simulink model "Stepper2"  (Simulink 7.6)
settings: Solver=ode45  StartTime=0.0  StopTime=1  RelTol=1e-3
libraries: simulink x13
settings Model: Creator=MTRStudent  LastModifiedBy=Mr_lex
settings DebuggingCC: StrictBusMsg=Warning

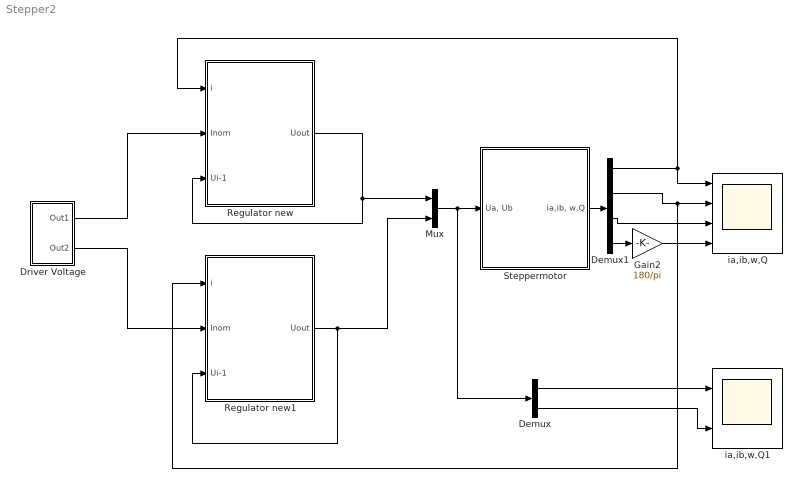
== system Stepper2 ==
  Demux : Demux  Outputs=2
  Demux1 : Demux
  Driver Voltage : Subsystem
  Gain2 : Gain  Gain=180/pi
  Mux : Mux  Inputs=2
  Regulator new : Subsystem
  Regulator new1 : Subsystem
  Steppermotor : Subsystem
  ia,ib,w,Q : Scope  NumInputPorts=4
      settings: TimeRange=0.004  YMin=-0.125~5.875~22~0.7  YMax=0.125~6.125~28.5~2.5  SaveName=ScopeData2
  ia,ib,w,Q1 : Scope  NumInputPorts=2
      settings: YMin=5.45~-2.75  YMax=6.4~1.25
  wires:
  Demux1/1 -> ia,ib,w,Q/1, Regulator new/1(i)
  Demux1/2 -> ia,ib,w,Q/2, Regulator new1/1(i)
  Demux1/3 -> ia,ib,w,Q/3
  Demux1/4 -> Gain2/1
  Steppermotor/1("ia,ib, w,Q") -> Demux1/1
  Mux/1 -> Steppermotor/1("Ua, Ub"), Demux/1
  Demux/1 -> ia,ib,w,Q1/1
  Demux/2 -> ia,ib,w,Q1/2
  Regulator new1/1(Uout) -> Mux/2, Regulator new1/3(Ui-1)
  Regulator new/1(Uout) -> Mux/1, Regulator new/3(Ui-1)
  Gain2/1 -> ia,ib,w,Q/4
  Driver Voltage/1(Out1) -> Regulator new/2(Inom)
  Driver Voltage/2(Out2) -> Regulator new1/2(Inom)

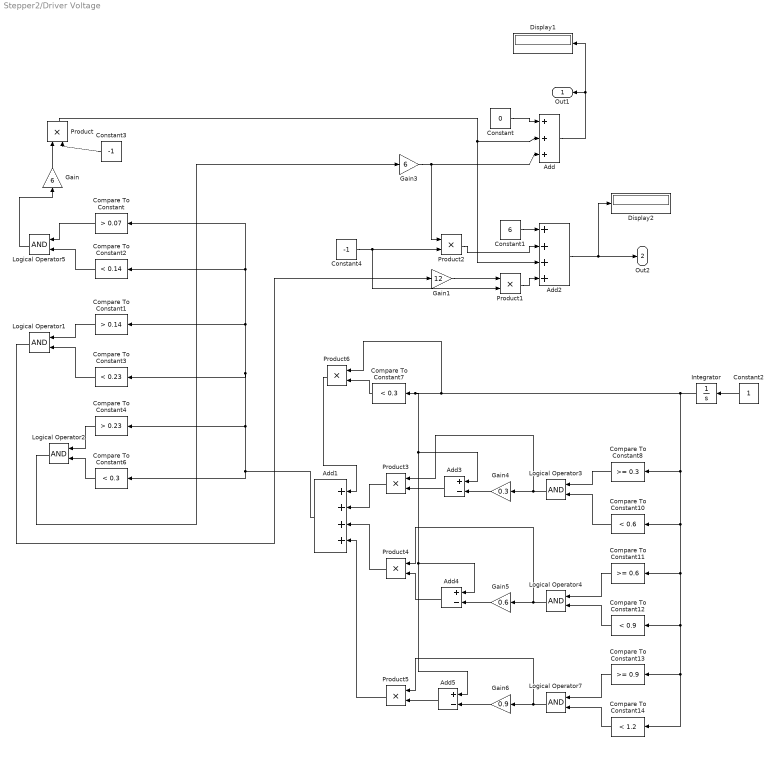
== system Stepper2/Driver Voltage ==
  Add : Sum  Inputs=+++
  Add1 : Sum  Inputs=++++
  Add2 : Sum  Inputs=++++
  Add3 : Sum  Inputs=+-
  Add4 : Sum  Inputs=+-
  Add5 : Sum  Inputs=+-
  Compare To Constant : simulink/Logic and Bit Operations/Compare To Constant  SystemSampleTime=-1  relop=>  const=0.07  LogicOutDataTypeMode=uint8  ZeroCross=off
  Compare To Constant1 : simulink/Logic and Bit Operations/Compare To Constant  SystemSampleTime=-1  relop=>  const=0.14  LogicOutDataTypeMode=uint8  ZeroCross=off
  Compare To Constant10 : simulink/Logic and Bit Operations/Compare To Constant  SystemSampleTime=-1  relop=<  const=0.6  LogicOutDataTypeMode=uint8  ZeroCross=off
  Compare To Constant11 : simulink/Logic and Bit Operations/Compare To Constant  SystemSampleTime=-1  relop=>=  const=0.6  LogicOutDataTypeMode=uint8  ZeroCross=off
  Compare To Constant12 : simulink/Logic and Bit Operations/Compare To Constant  SystemSampleTime=-1  relop=<  const=0.9  LogicOutDataTypeMode=uint8  ZeroCross=off
  Compare To Constant13 : simulink/Logic and Bit Operations/Compare To Constant  SystemSampleTime=-1  relop=>=  const=0.9  LogicOutDataTypeMode=uint8  ZeroCross=off
  Compare To Constant14 : simulink/Logic and Bit Operations/Compare To Constant  SystemSampleTime=-1  relop=<  const=1.2  LogicOutDataTypeMode=uint8  ZeroCross=off
  Compare To Constant2 : simulink/Logic and Bit Operations/Compare To Constant  SystemSampleTime=-1  relop=<  const=0.14  LogicOutDataTypeMode=uint8  ZeroCross=off
  Compare To Constant3 : simulink/Logic and Bit Operations/Compare To Constant  SystemSampleTime=-1  relop=<  const=0.23  LogicOutDataTypeMode=uint8  ZeroCross=off
  Compare To Constant4 : simulink/Logic and Bit Operations/Compare To Constant  SystemSampleTime=-1  relop=>  const=0.23  LogicOutDataTypeMode=uint8  ZeroCross=off
  Compare To Constant6 : simulink/Logic and Bit Operations/Compare To Constant  SystemSampleTime=-1  relop=<  const=0.3  LogicOutDataTypeMode=uint8  ZeroCross=off
  Compare To Constant7 : simulink/Logic and Bit Operations/Compare To Constant  SystemSampleTime=-1  relop=<  const=0.3  LogicOutDataTypeMode=uint8  ZeroCross=off
  Compare To Constant8 : simulink/Logic and Bit Operations/Compare To Constant  SystemSampleTime=-1  relop=>=  const=0.3  LogicOutDataTypeMode=uint8  ZeroCross=off
  Constant : Constant  Value=0
  Constant1 : Constant  Value=6
  Constant2 : Constant
  Constant3 : Constant  Value=-1
  Constant4 : Constant  Value=-1
  Display1 : Display
  Display2 : Display
  Gain : Gain  Gain=6
  Gain1 : Gain  Gain=12
  Gain3 : Gain  Gain=6
  Gain4 : Gain  Gain=0.3
  Gain5 : Gain  Gain=0.6
  Gain6 : Gain  Gain=0.9
  Integrator : Integrator
  Logical Operator{1..5,7} (6 alike) : Logic  AllPortsSameDT=off  OutDataTypeStr=boolean
  Product{,1..6} (7 alike) : Product  RndMeth=Zero
  Out1 : Outport
  Out2 : Outport  Port=2
  wires:
  Add/1 -> Out1/1, Display1/1
  Constant/1 -> Add/1
  Constant1/1 -> Add2/1
  Gain/1 -> Product/1
  Constant3/1 -> Product/2
  Compare To Constant/1 -> Logical Operator5/1
  Compare To Constant2/1 -> Logical Operator5/2
  Logical Operator5/1 -> Gain/1
  Gain1/1 -> Product1/1
  Product1/1 -> Add2/4
  Compare To Constant1/1 -> Logical Operator1/1
  Compare To Constant3/1 -> Logical Operator1/2
  Gain3/1 -> Add/3, Product2/1
  Product2/1 -> Add2/2
  Add2/1 -> Out2/1, Display2/1
  Product/1 -> Add/2, Add2/3
  Constant4/1 -> Product2/2, Product1/2
  Logical Operator1/1 -> Gain1/1
  Compare To Constant4/1 -> Logical Operator2/1
  Compare To Constant6/1 -> Logical Operator2/2
  Logical Operator2/1 -> Gain3/1
  Constant2/1 -> Integrator/1
  Integrator/1 -> Compare To Constant8/1, Compare To Constant10/1, Compare To Constant11/1, Compare To Constant12/1, Compare To Constant13/1, Compare To Constant14/1, Add4/1, Add5/1, Add3/1, Compare To Constant7/1, Product6/1
  Compare To Constant8/1 -> Logical Operator3/1
  Compare To Constant10/1 -> Logical Operator3/2
  Compare To Constant11/1 -> Logical Operator4/1
  Compare To Constant12/1 -> Logical Operator4/2
  Compare To Constant13/1 -> Logical Operator7/1
  Compare To Constant14/1 -> Logical Operator7/2
  Logical Operator3/1 -> Gain4/1, Product3/1
  Logical Operator4/1 -> Gain5/1, Product4/1
  Logical Operator7/1 -> Gain6/1, Product5/1
  Gain6/1 -> Add5/2
  Gain5/1 -> Add4/2
  Gain4/1 -> Add3/2
  Add1/1 -> Compare To Constant/1, Compare To Constant2/1, Compare To Constant1/1, Compare To Constant3/1, Compare To Constant4/1, Compare To Constant6/1
  Product6/1 -> Add1/1
  Compare To Constant7/1 -> Product6/2
  Add3/1 -> Product3/2
  Product3/1 -> Add1/2
  Add4/1 -> Product4/2
  Product4/1 -> Add1/3
  Add5/1 -> Product5/2
  Product5/1 -> Add1/4

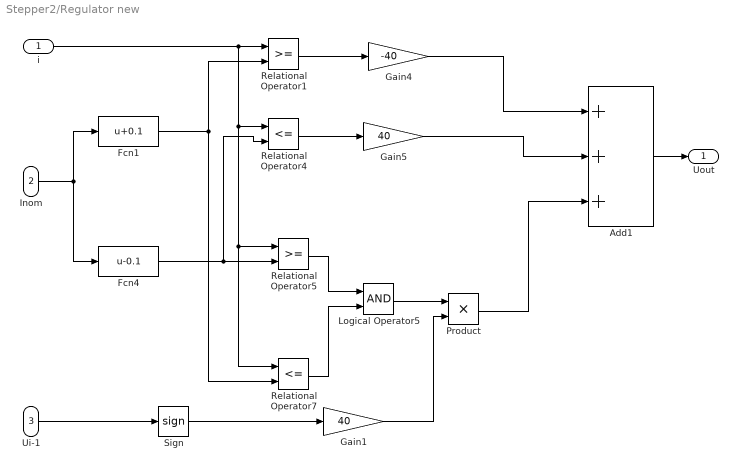
== system Stepper2/Regulator new ==
  i : Inport
  Inom : Inport  Port=2
  Ui-1 : Inport  Port=3
  Add1 : Sum  Inputs=+++  OutDataTypeStr=double
  Fcn1 : Fcn  Expr=u+0.1
  Fcn4 : Fcn  Expr=u-0.1
  Gain1 : Gain  Gain=40
  Gain4 : Gain  Gain=-40
  Gain5 : Gain  Gain=40
  Logical Operator5 : Logic  AllPortsSameDT=off  OutDataTypeStr=boolean
  Product : Product  RndMeth=Zero
  Relational Operator1 : RelationalOperator  OutDataTypeStr=boolean  ZeroCross=off
  Relational Operator4 : RelationalOperator  Operator=<=  OutDataTypeStr=boolean  ZeroCross=off
  Relational Operator5 : RelationalOperator  OutDataTypeStr=boolean  ZeroCross=off
  Relational Operator7 : RelationalOperator  Operator=<=  OutDataTypeStr=boolean  ZeroCross=off
  Sign : Signum
  Uout : Outport
  wires:
  Logical Operator5/1 -> Product/1
  Product/1 -> Add1/3
  Add1/1 -> Uout/1
  Ui-1/1 -> Sign/1
  Relational Operator7/1 -> Logical Operator5/2
  Relational Operator5/1 -> Logical Operator5/1
  Gain5/1 -> Add1/2
  Gain4/1 -> Add1/1
  Relational Operator4/1 -> Gain5/1
  Fcn4/1 -> Relational Operator5/2, Relational Operator4/2
  Relational Operator1/1 -> Gain4/1
  Fcn1/1 -> Relational Operator7/2, Relational Operator1/2
  i/1 -> Relational Operator7/1, Relational Operator5/1, Relational Operator4/1, Relational Operator1/1
  Inom/1 -> Fcn1/1, Fcn4/1
  Sign/1 -> Gain1/1
  Gain1/1 -> Product/2

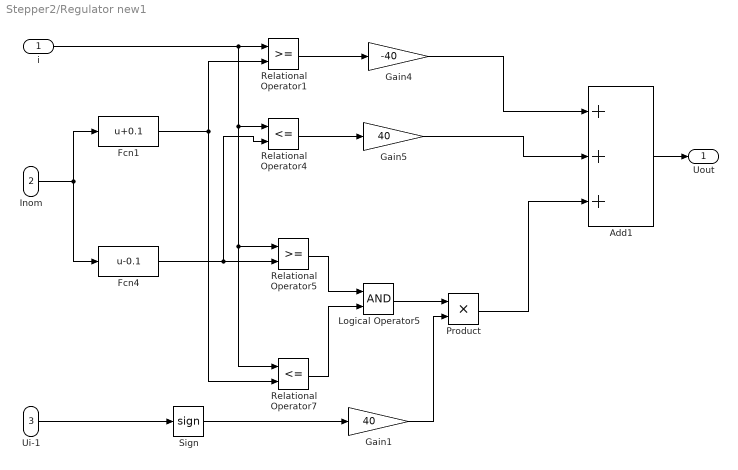
== system Stepper2/Regulator new1 ==
  i : Inport
  Inom : Inport  Port=2
  Ui-1 : Inport  Port=3
  Add1 : Sum  Inputs=+++  OutDataTypeStr=double
  Fcn1 : Fcn  Expr=u+0.1
  Fcn4 : Fcn  Expr=u-0.1
  Gain1 : Gain  Gain=40
  Gain4 : Gain  Gain=-40
  Gain5 : Gain  Gain=40
  Logical Operator5 : Logic  AllPortsSameDT=off  OutDataTypeStr=boolean
  Product : Product  RndMeth=Zero
  Relational Operator1 : RelationalOperator  OutDataTypeStr=boolean  ZeroCross=off
  Relational Operator4 : RelationalOperator  Operator=<=  OutDataTypeStr=boolean  ZeroCross=off
  Relational Operator5 : RelationalOperator  OutDataTypeStr=boolean  ZeroCross=off
  Relational Operator7 : RelationalOperator  Operator=<=  OutDataTypeStr=boolean  ZeroCross=off
  Sign : Signum
  Uout : Outport
  wires:
  Inom/1 -> Fcn4/1, Fcn1/1
  i/1 -> Relational Operator1/1, Relational Operator4/1, Relational Operator5/1, Relational Operator7/1
  Fcn1/1 -> Relational Operator1/2, Relational Operator7/2
  Relational Operator1/1 -> Gain4/1
  Fcn4/1 -> Relational Operator4/2, Relational Operator5/2
  Relational Operator4/1 -> Gain5/1
  Gain4/1 -> Add1/1
  Gain5/1 -> Add1/2
  Relational Operator5/1 -> Logical Operator5/1
  Relational Operator7/1 -> Logical Operator5/2
  Ui-1/1 -> Sign/1
  Add1/1 -> Uout/1
  Product/1 -> Add1/3
  Logical Operator5/1 -> Product/1
  Gain1/1 -> Product/2
  Sign/1 -> Gain1/1

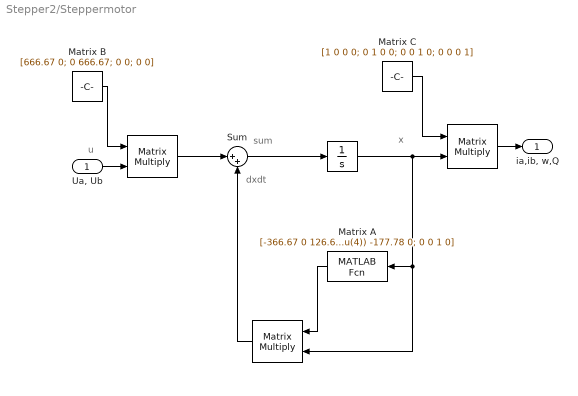
== system Stepper2/Steppermotor ==
  note: x
  note: dxdt
  note: sum
  note: u
  "Ua, Ub" : Inport
  " " : Integrator
  "  " : Product  Multiplication=Matrix(*)  RndMeth=Zero
  "    " : Product  Multiplication=Matrix(*)  RndMeth=Zero
  "         " : Product  Multiplication=Matrix(*)  RndMeth=Zero
  Matrix A : MATLABFcn  MATLABFcn=[-366.67 0 126.67*sin(50*u(4)) 0; 0 -366.67 126.67*cos(50*u(4)) 0; -4222.22*sin(50*u(4)) 4222.22*cos(50*u(4)) -177.78 0; 0 0 1 0]  Output1D=off
  Matrix B : Constant  Value=[666.67 0; 0 666.67; 0 0; 0 0]
  Matrix C : Constant  Value=[1 0 0 0; 0 1 0 0; 0 0 1 0; 0 0 0 1]
  Sum : Sum  Inputs=|++
  "ia,ib, w,Q" : Outport
  wires:
  " "/1 -> "    "/2, Matrix A/1, "  "/2
  Sum/1 -> " "/1
  Matrix C/1 -> "    "/1
  Matrix B/1 -> "         "/1
  "         "/1 -> Sum/1
  "  "/1 -> Sum/2
  Matrix A/1 -> "  "/1
  "    "/1 -> "ia,ib, w,Q"/1
  "Ua, Ub"/1 -> "         "/2
